simulink model "Aufgabe3_simu"  (Simulink 9.2)
settings: Solver=VariableStepAuto  StartTime=0.0  StopTime=10.0  RelTol=1e-3
libraries: simulink x4
settings Model: Creator=danial  LastModifiedBy=danial
settings DataIOCC: LimitDataPoints=off  SaveFormat=Dataset  SignalLoggingSaveFormat=Dataset
settings OptimizationCC: LifeSpan=auto
settings DebuggingCC: UnderspecifiedInitializationDetection=Simplified  MergeDetectMultiDrivingBlocksExec=error  FcnCallInpInsideContextMsg=error  StateNameClashWarn=none  SFUnexpectedBacktrackingDiag=error  SFNoUnconditionalDefaultTransitionDiag=error  SFExecutionAtInitializationDiag=warning
settings HardwareCC: ProdBitPerPointer=64  ProdBitPerSizeT=64  ProdBitPerPtrDiffT=64  ProdLargestAtomicFloat=Float  ProdIntDivRoundTo=Zero  ProdEndianess=LittleEndian  ProdWordSize=64  ProdHWDeviceType=Intel->x86-64 (Windows64)
settings ModelReferenceCC: PropagateSignalLabelsOutOfModel=on
settings SFSimCC: SimUseLocalCustomCode=on
settings RTWCC: RTWUseLocalCustomCode=on
settings CodeAppCC: StateflowObjectComments=off
settings GRTTargetCC: TargetLangStandard=C99 (ISO)  GeneratePreprocessorConditionals=Use local settings  CombineOutputUpdateFcns=on  GRTInterface=off
settings ConfigComp: CovMetricSettings=dwe  CovHtmlReporting=off  CovSaveCumulativeToWorkspaceVar=off  CovSaveSingleToWorkspaceVar=off  CovExternalEMLEnable=on

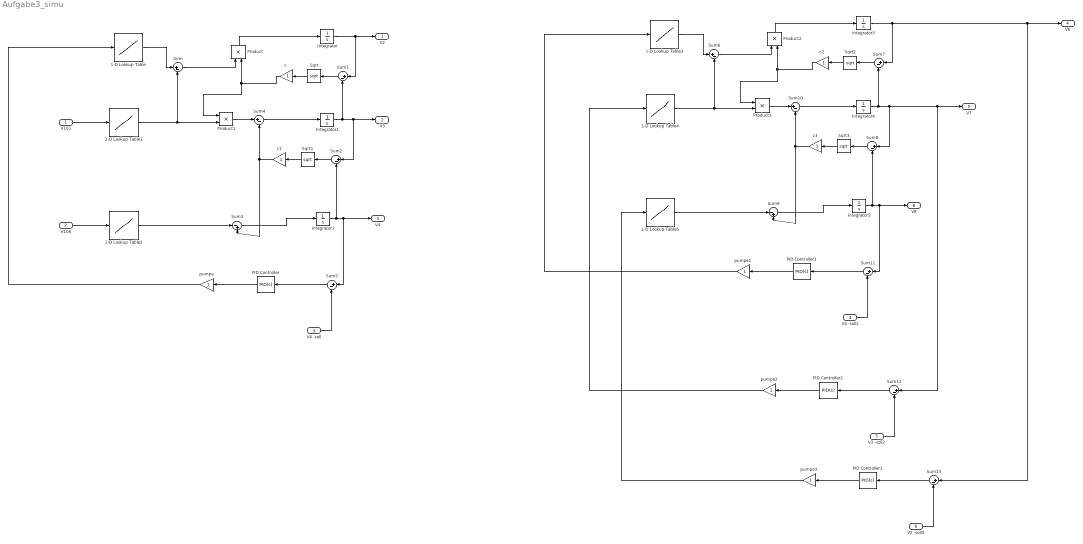
== system Aufgabe3_simu ==
  V101 : Inport
  V106 : Inport  Port=2
  V4 -soll : Inport  Port=3
  V4 -soll1 : Inport  Port=4
  V3 -soll2 : Inport  Port=5
  V2 -soll3 : Inport  Port=6
  1-D Lookup Table{,1..5} (6 alike) : Lookup_n-D  NumberOfTableDimensions=1  BreakpointsForDimension1=[-5:5]  Table=tanh([-5:5])  InternalRulePriority=Speed  RndMeth=Simplest  InputSameDT=on
  Integrator{,1..5} (6 alike) : Integrator
  PID Controller{,1..3} (4 alike) : simulink/Continuous/PID Controller  Controller=PID  Form=Parallel  TimeDomain=Continuous-time  SampleTime=-1  IntegratorMethod=Forward Euler  FilterMethod=Forward Euler  ControllerParametersSource=internal  P=1  I=1  D=0  UseFilter=on  N=100  TunerSelectOption=Transfer Function Based (PID Tuner App)  InitialConditionSource=internal  InitialConditionForIntegrator=0  InitialConditionForFilter=0  DifferentiatorICPrevScaledInput=0  ExternalReset=none  TrackingMode=off  Kt=1  LimitOutput=off  UpperSaturationLimit=inf  LowerSaturationLimit=-inf  LinearizeAsGain=on  AntiWindupMode=none  Kb=1  POutMin=[]  POutMax=[]  IOutMin=[]  IOutMax=[]  DOutMin=[]  DOutMax=[]  NOutMin=[]  NOutMax=[]  SumOutMin=[]  SumOutMax=[]  SaturationOutMin=[]  SaturationOutMax=[]  PParamMin=[]  PParamMax=[]  IParamMin=[]  IParamMax=[]  DParamMin=[]  DParamMax=[]  NParamMin=[]  NParamMax=[]  KbParamMin=[]  KbParamMax=[]  KtParamMin=[]  KtParamMax=[]  KbOutMin=[]  KbOutMax=[]  KtOutMin=[]  KtOutMax=[]  IntegratorOutMin=[]  IntegratorOutMax=[]  FilterOutMin=[]  FilterOutMax=[]  SumI1OutMin=[]  SumI1OutMax=[]  SumI2OutMin=[]  SumI2OutMax=[]  SumI3OutMin=[]  SumI3OutMax=[]  SumI4OutMin=[]  SumI4OutMax=[]  SumDOutMin=[]  SumDOutMax=[]  DifferentiatorOutMin=[]  DifferentiatorOutMax=[]  FilterDiffOutCoefMin=[]  FilterDiffOutCoefMax=[]  ReciprocalOutMin=[]  ReciprocalOutMax=[]  SumDenOutMin=[]  SumDenOutMax=[]  SumNumOutMin=[]  SumNumOutMax=[]  DivideOutMin=[]  DivideOutMax=[]  IntegratorContinuousStateAttributes=''  IntegratorStateMustResolveToSignalObject=off  IntegratorRTWStateStorageClass=Auto  FilterContinuousStateAttributes=''  FilterStateMustResolveToSignalObject=off  FilterRTWStateStorageClass=Auto  ParallelPVariant=InternalParameters  IdealPVariant=Disabled  IVariant=InternalParameters  DVariant=InternalParameters  IntegratorVariant=Continuous  SatVariant=Disabled  AWVariant=Passthrough  PCopyVariant=Disabled  TRVariant=Disabled  FdbkBlocksVariant=Forward  IdealPFdbkVariant=Disabled  SatFdbkVariant=Disabled  DerivativeFilterVariant=ContFilter  NVariant=InternalParameters  NCopyVariant=Disabled  FilterICVariant=InternalICsFilter  IntegratorICVariant=InternalICs  ExternalResetVariant=Disabled  TRSumVariant=Passthrough  SumFdbkVariant=Disabled  SumVariant=Sum_PID
  Product{,1..3} (4 alike) : Product
  Sqrt{,1..3} (4 alike) : Sqrt  SaturateOnIntegerOverflow=on
  Sum{,1..2,4..8,10..13} (12 alike) : Sum  Inputs=|+-
  Sum3 : Sum  Inputs=|-+
  Sum9 : Sum  Inputs=|-+
  c{,1..3} (4 alike) : Gain
  pumpe{,1..3} (4 alike) : Gain
  V2 : Outport
  V3 : Outport  Port=2
  V4 : Outport  Port=3
  V6 : Outport  Port=4
  V7 : Outport  Port=5
  V8 : Outport  Port=6
  wires:
  pumpe/1 -> 1-D Lookup Table/1
  1-D Lookup Table/1 -> Sum/1
  V101/1 -> 1-D Lookup Table1/1
  V106/1 -> 1-D Lookup Table2/1
  1-D Lookup Table1/1 -> Product1/2, Sum/2
  Integrator/1 -> Sum1/1, V2/1
  Sum1/1 -> Sqrt/1
  Sqrt/1 -> c/1
  Sum/1 -> Product/1
  c/1 -> Product1/1, Product/2
  Product/1 -> Integrator/1
  Integrator1/1 -> Sum1/2, Sum2/1, V3/1
  Integrator2/1 -> Sum5/1, V4/1, Sum2/2
  Sum2/1 -> Sqrt1/1
  Sqrt1/1 -> c1/1
  1-D Lookup Table2/1 -> Sum3/1
  c1/1 -> Sum3/2, Sum4/2
  Sum3/1 -> Integrator2/1
  Sum4/1 -> Integrator1/1
  Product1/1 -> Sum4/1
  PID Controller/1 -> pumpe/1
  Sum5/1 -> PID Controller/1
  V4 -soll/1 -> Sum5/2
  Sum8/1 -> Sqrt3/1
  Sqrt2/1 -> c2/1
  c3/1 -> Sum9/2, Sum10/2
  Sqrt3/1 -> c3/1
  Integrator4/1 -> Sum7/2, Sum8/1, Sum12/1, V7/1
  Sum7/1 -> Sqrt2/1
  Product2/1 -> Integrator3/1
  Product3/1 -> Sum10/1
  Sum9/1 -> Integrator5/1
  1-D Lookup Table5/1 -> Sum9/1
  1-D Lookup Table4/1 -> Product3/2, Sum6/2
  c2/1 -> Product3/1, Product2/2
  Sum6/1 -> Product2/1
  Sum10/1 -> Integrator4/1
  1-D Lookup Table3/1 -> Sum6/1
  PID Controller1/1 -> pumpe1/1
  pumpe1/1 -> 1-D Lookup Table3/1
  V4 -soll1/1 -> Sum11/2
  Sum11/1 -> PID Controller1/1
  Integrator5/1 -> Sum11/1, V8/1, Sum8/2
  pumpe2/1 -> 1-D Lookup Table4/1
  V3 -soll2/1 -> Sum12/2
  PID Controller2/1 -> pumpe2/1
  Sum12/1 -> PID Controller2/1
  V2 -soll3/1 -> Sum13/2
  pumpe3/1 -> 1-D Lookup Table5/1
  PID Controller3/1 -> pumpe3/1
  Integrator3/1 -> Sum7/1, Sum13/1, V6/1
  Sum13/1 -> PID Controller3/1
